simulink subsystem "PlantPModel"  (R2020b)
settings: Solver=VariableStepAuto  StartTime=0.0  StopTime=10.0  RelTol=1e-3
settings Model: Creator=Stend  LastModifiedBy=Stend

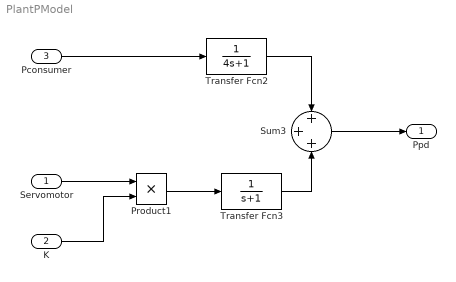
== system PlantPModel ==
  Servomotor : Inport
  K : Inport  Port=2
  Pconsumer : Inport  Port=3
  Product1 : Product
  Sum3 : Sum  Inputs=+++  InputSameDT=on  SaturateOnIntegerOverflow=on  OutDataTypeStr=Inherit: Same as first input
  Transfer Fcn2 : TransferFcn  Denominator=[4 1]
  Transfer Fcn3 : TransferFcn  Denominator=[1 1]
  Ppd : Outport
  wires:
  Sum3/1 -> Ppd/1
  Transfer Fcn2/1 -> Sum3/1
  Servomotor/1 -> Product1/1
  K/1 -> Product1/2
  Product1/1 -> Transfer Fcn3/1
  Pconsumer/1 -> Transfer Fcn2/1
  Transfer Fcn3/1 -> Sum3/3
